simulink library "HIL_GenSet"  (Simulink 7.8)
settings: Solver=ode45  StartTime=0.0  StopTime=10.0  RelTol=1e-3
values from neighbouring files (symbols this model uses):
  Ts = 80e-6    (= 8e-05)    [global_parameters.m]    (also in scopeBuffer.m)
undefined symbols (not defined in the file or in its folder): DiscIntNeverNeededParam, Ts_Power
libraries: simulink x77, powerlib x55, discretizing x28
(part 6 of 9)

== system HIL_GenSet/GenSet_3p5MW_nPID_Manual_RTLAB/Generator with  Primary Controllers/72.5 kva Diesel Engine Speed & Voltage Control fast/IEEE GOVERNOR & DIESEL ENGINE ==
  note: ACTUATOR
  wref (pu) : Inport
  w (pu) : Inport  Port=2
  Reset : Inport  Port=3
  Discrete PID Controller : simulink/Continuous/PID Controller  Controller=PD  TimeDomain=Discrete-time  SampleTime=-1  IntegratorMethod=Forward Euler  FilterMethod=Forward Euler  Form=Parallel  P=1  I=0  D=0.5  N=10000  InitialConditionSource=internal  InitialConditionForIntegrator=0  InitialConditionForFilter=0  ExternalReset=either  ZeroCross=off  LimitOutput=off  UpperSaturationLimit=.5  LowerSaturationLimit=-.5  LinearizeAsGain=off  AntiWindupMode=none  Kb=1  TrackingMode=off  Kt=1  PParamMin=[]  PParamMax=[]  IParamMin=[]  IParamMax=[]  DParamMin=[]  DParamMax=[]  NParamMin=[]  NParamMax=[]  KbParamMin=[]  KbParamMax=[]  KtParamMin=[]  KtParamMax=[]  POutMin=[]  POutMax=[]  IOutMin=[]  IOutMax=[]  DOutMin=[]  DOutMax=[]  NOutMin=[]  NOutMax=[]  KbOutMin=[]  KbOutMax=[]  KtOutMin=[]  KtOutMax=[]  IntegratorOutMin=[]  IntegratorOutMax=[]  FilterOutMin=[]  FilterOutMax=[]  SumOutMin=[]  SumOutMax=[]  SumI1OutMin=[]  SumI1OutMax=[]  SumI2OutMin=[]  SumI2OutMax=[]  SumI3OutMin=[]  SumI3OutMax=[]  SumDOutMin=[]  SumDOutMax=[]  SaturationOutMin=[]  SaturationOutMax=[]  IntegratorContinuousStateAttributes=''  IntegratorStateMustResolveToSignalObject=off  IntegratorRTWStateStorageClass=Auto  FilterContinuousStateAttributes=''  FilterStateMustResolveToSignalObject=off  FilterRTWStateStorageClass=Auto
  Discrete-Time Integrator : DiscreteIntegrator  IntegratorMethod=Integration: Backward Euler  ExternalReset=either  InitialCondition=Pm0  SampleTime=-1  LimitOutput=on  UpperSaturationLimit=Tlim(2)  LowerSaturationLimit=Tlim(1)  ICPrevOutput=DiscIntNeverNeededParam  ICPrevScaledInput=DiscIntNeverNeededParam
  ENGINE Td : TransportDelay  DelayTime=Td  InitialOutput=Pm0  BufferSize=7168
  Gain K : Gain  Gain=K  SaturateOnIntegerOverflow=on  OutDataTypeStr=Inherit: Same as input  ParamDataTypeStr=Inherit: Same as input
  Product : Product  SaturateOnIntegerOverflow=on  InputSameDT=on  OutDataTypeStr=Inherit: Same as first input
  Sum : Sum  Inputs=+-  SaturateOnIntegerOverflow=on  InputSameDT=on  OutDataTypeStr=Inherit: Same as first input
  TF3 : discretizing/Discretized Transfer Fcn  Numerator=1  Denominator=([Ta(3) 1])  AbsTol=auto  SampleTime=Ts  method=zoh  Wc=1
  TF4 : discretizing/Discretized Transfer Fcn  Numerator=([Ta(1) 1])  Denominator=([Ta(2) 1])  AbsTol=auto  SampleTime=Ts  method=zoh  Wc=1
  Pmec (pu) : Outport
  wires:
  Reset/1 -> Discrete PID Controller/2, Discrete-Time Integrator/2
  TF4/1 -> TF3/1
  TF3/1 -> Discrete-Time Integrator/1
  Discrete-Time Integrator/1 -> ENGINE Td/1  "Torque"
  Product/1 -> Pmec (pu)/1
  wref (pu)/1 -> Sum/1
  ENGINE Td/1 -> Product/1
  w (pu)/1 -> Sum/2, Product/2
  Discrete PID Controller/1 -> Gain K/1
  Sum/1 -> Discrete PID Controller/1
  Gain K/1 -> TF4/1

== system HIL_GenSet/GenSet_3p5MW_new_PID_RTLAB/60kW Generator with  Primary Controllers/72.5 kva Diesel Engine Speed & Voltage Control fast/GOVERNOR & DIESEL ENGINE1 ==
  note: ACTUATOR
  wref (pu) : Inport
  w (pu) : Inport  Port=2
  Reset : Inport  Port=3
  Discrete PID Controller : simulink/Continuous/PID Controller  Controller=PD  TimeDomain=Discrete-time  SampleTime=-1  IntegratorMethod=Forward Euler  FilterMethod=Forward Euler  Form=Parallel  P=1  I=0  D=0.5  N=10000  InitialConditionSource=internal  InitialConditionForIntegrator=0  InitialConditionForFilter=0  ExternalReset=either  ZeroCross=off  LimitOutput=off  UpperSaturationLimit=.5  LowerSaturationLimit=-.5  LinearizeAsGain=off  AntiWindupMode=none  Kb=1  TrackingMode=off  Kt=1  PParamMin=[]  PParamMax=[]  IParamMin=[]  IParamMax=[]  DParamMin=[]  DParamMax=[]  NParamMin=[]  NParamMax=[]  KbParamMin=[]  KbParamMax=[]  KtParamMin=[]  KtParamMax=[]  POutMin=[]  POutMax=[]  IOutMin=[]  IOutMax=[]  DOutMin=[]  DOutMax=[]  NOutMin=[]  NOutMax=[]  KbOutMin=[]  KbOutMax=[]  KtOutMin=[]  KtOutMax=[]  IntegratorOutMin=[]  IntegratorOutMax=[]  FilterOutMin=[]  FilterOutMax=[]  SumOutMin=[]  SumOutMax=[]  SumI1OutMin=[]  SumI1OutMax=[]  SumI2OutMin=[]  SumI2OutMax=[]  SumI3OutMin=[]  SumI3OutMax=[]  SumDOutMin=[]  SumDOutMax=[]  SaturationOutMin=[]  SaturationOutMax=[]  IntegratorContinuousStateAttributes=''  IntegratorStateMustResolveToSignalObject=off  IntegratorRTWStateStorageClass=Auto  FilterContinuousStateAttributes=''  FilterStateMustResolveToSignalObject=off  FilterRTWStateStorageClass=Auto
  Discrete-Time Integrator : DiscreteIntegrator  IntegratorMethod=Integration: Backward Euler  ExternalReset=either  InitialCondition=Pm0  SampleTime=Ts_Power  LimitOutput=on  UpperSaturationLimit=Tlim(2)  LowerSaturationLimit=Tlim(1)  ICPrevOutput=DiscIntNeverNeededParam  ICPrevScaledInput=DiscIntNeverNeededParam
  ENGINE Td : TransportDelay  DelayTime=Td  InitialOutput=Pm0  BufferSize=7168
  Gain K : Gain  Gain=K  SaturateOnIntegerOverflow=on  OutDataTypeStr=Inherit: Same as input  ParamDataTypeStr=Inherit: Same as input
  Product : Product  SaturateOnIntegerOverflow=on  InputSameDT=on  OutDataTypeStr=Inherit: Same as first input
  Scope : Scope  NumInputPorts=2
      settings: YMin=-1~-1  YMax=2~2  SaveName=ScopeData20
  Sum : Sum  Inputs=+-  SampleTime=Ts_Power  SaturateOnIntegerOverflow=on  InputSameDT=on  OutDataTypeStr=Inherit: Same as first input
  TF3 : discretizing/Discretized Transfer Fcn  Numerator=1  Denominator=([Ta(3) 1])  AbsTol=auto  SampleTime=Ts_Power  method=zoh  Wc=1
  TF4 : discretizing/Discretized Transfer Fcn  Numerator=([Ta(1) 1])  Denominator=([Ta(2) 1])  AbsTol=auto  SampleTime=Ts_Power  method=zoh  Wc=1
  Pmec (pu) : Outport
  wires:
  Reset/1 -> Discrete PID Controller/2, Discrete-Time Integrator/2
  TF4/1 -> TF3/1
  TF3/1 -> Discrete-Time Integrator/1
  Discrete-Time Integrator/1 -> Scope/2, ENGINE Td/1  "Torque"
  Product/1 -> Scope/1, Pmec (pu)/1
  wref (pu)/1 -> Sum/1
  ENGINE Td/1 -> Product/1
  w (pu)/1 -> Sum/2, Product/2
  Discrete PID Controller/1 -> Gain K/1
  Sum/1 -> Discrete PID Controller/1
  Gain K/1 -> TF4/1

== system HIL_GenSet/GenSet_3p5MW_new_PID_RTLAB/60kW Generator with  Primary Controllers/72.5 kva Diesel Engine Speed & Voltage Control fast/Subsystem ==
  note: link disabled
  note: link disabled
  vref : Inport
  v : Inport  Port=2
  vstab : Inport  Port=3
  Damping kf.s / (tf.s +1) : Subsystem
  Exciter  1 / (te.s + ke) : Subsystem
  Lead Lag Compensator tc.s+1 / tb.s+1 : Subsystem  AncestorBlock=|  mask(Discrete Lead-Lag Controller){T1=tgr(2), T2=tgr(1), V_Init=exc(1)*v0(2)/reg(1), Ts=Ts}
      | powerlib_extras/Discrete 
      | Control Blocks/Discrete
      | Lead-Lag
      mask prompts: T1 "Time constant T1 (s):"; T2 "Time constant T2 (s):"; V_Init "Initial input and output:"; Ts "Sample time (s):"
      mask help:
      | This block implements a discrete lead-lag controller:
      |
      |          1+T1s
      | H(s)= ------
      |          1+T2s
      |
      | States are initialized according to initial input anf output value so that simulation starts in steady state.
      mask init: same as HIL_GenSet/GenSet_3p5MW_RTLAB/60kW Generator with  Primary Controllers/72.5 kva Diesel Engine Speed & Voltage Control fast/Subsystem/Lead Lag Compensator tc.s+1 / tb.s+1
      mask Display: disp('1+T1s\n---\n1+T2s')
  Low Pass Filter 1 / (tr.s +1) (with IC) : Subsystem  AncestorBlock=|  mask(Discrete 1st-Order Filter){FilterType=Lowpass, Tc=tr, Ts=Ts, Initialize=on, Vac_Init=[0 0 60], Vdc_Init=v0(1), PlotResponse=off, param1=[1 500 0.1]}
      | powerlib_extras/Discrete 
      | Control Blocks/Discrete
      | 1st-Order
      | Discrete Filter
      mask prompts: FilterType "Filter Type:"; Tc "Time constant (s):"; Ts "Sample time:"; Initialize "Initialize filter states"; Vac_Init "AC initial input: [ Mag  Phase(degrees)  Freq(Hz) ]"; Vdc_Init "DC Initial input:"; PlotResponse "Plot filter response"; param1 "Frequency range(Hz) : [Start  End  Inc.]"
      mask init: same as HIL_GenSet/GenSet_3p5MW_RTLAB/60kW Generator with  Primary Controllers/72.5 kva Diesel Engine Speed & Voltage Control fast/Subsystem/Low Pass Filter 1 / (tr.s +1) (with IC)
      mask StyleString: popup(Lowpass|Highpass),edit,edit,checkbox,edit,edit,checkbox,edit
      mask CallbackString: |||p4=get_param(gcb,'Initialize');if strcmp(p4,'on');visible={'on','on','on','on','on','on','on',get_param(gcb,'PlotResponse')};else;visible={'on','on','on','on','off','off','on',get_param(gcb,'PlotResponse')};end;set_param(gcb,'MaskVisibilities',visible)|||p7=get_param(gcb,'PlotResponse');if strcmp(p7,'on');visible={'on','on','on','on',get_param(gcb,'Initialize'),get_param(gcb,'Initialize'),'on','on'};else;visible={'on','on','on','on',get_param(gcb,'Initialize'),get_param(gcb,'Initialize'),'on','off'};end;set_param(gcb,'MaskVisibilities',visible)|
      mask Display: plot(X,Y);
  Main Regulator ka / (ta.s +1) : Subsystem
  Sum : Sum  Inputs=++-+-  SaturateOnIntegerOverflow=on  InputSameDT=on  OutDataTypeStr=Inherit: Same as first input
  Unit Delay1 : UnitDelay  SampleTime=Ts
  Unit Delay2 : UnitDelay  X0=v0(2)  SampleTime=Ts
  Vf0 / ka : Constant  Value=v0(2)/reg(1)
  proportional saturation : Subsystem
  Vf1 : Outport  InitialOutput=0
  wires:
  Unit Delay2/1 -> Vf1/1
  Unit Delay1/1 -> Sum/5
  proportional saturation/1(Ef) -> Exciter  1 / (te.s + ke)/1(In)
  Lead Lag Compensator tc.s+1 / tb.s+1/1(Out1) -> Main Regulator ka / (ta.s +1)/1(In)
  Sum/1 -> Lead Lag Compensator tc.s+1 / tb.s+1/1(In1)
  v/1 -> Low Pass Filter 1 / (tr.s +1) (with IC)/1(In)
  vref/1 -> Sum/1
  vstab/1 -> Sum/4
  Low Pass Filter 1 / (tr.s +1) (with IC)/1(Out) -> proportional saturation/2(Vtf), Sum/3
  Vf0 / ka/1 -> Sum/2
  Main Regulator ka / (ta.s +1)/1(Out) -> proportional saturation/1(Efd)
  Damping kf.s / (tf.s +1)/1(Out) -> Unit Delay1/1
  Exciter  1 / (te.s + ke)/1(Out) -> Unit Delay2/1, Damping kf.s / (tf.s +1)/1(In)

== system HIL_GenSet/GenSet_4MW_14kV/Generator with  Primary Controllers/72.5 kva Diesel Engine Speed & Voltage Control fast/IEEE Excitation ==
  note: link disabled
  note: link disabled
  vref : Inport
  v : Inport  Port=2
  vstab : Inport  Port=3
  Damping kf.s / (tf.s +1) : Subsystem
  Exciter  1 / (te.s + ke) : Subsystem
  Lead Lag Compensator tc.s+1 / tb.s+1 : Subsystem  AncestorBlock=|  mask(Discrete Lead-Lag Controller){T1=tgr(2), T2=tgr(1), V_Init=exc(1)*v0(2)/reg(1), Ts=Ts}
      | powerlib_extras/Discrete 
      | Control Blocks/Discrete
      | Lead-Lag
      mask prompts: T1 "Time constant T1 (s):"; T2 "Time constant T2 (s):"; V_Init "Initial input and output:"; Ts "Sample time (s):"
      mask help:
      | This block implements a discrete lead-lag controller:
      |
      |          1+T1s
      | H(s)= ------
      |          1+T2s
      |
      | States are initialized according to initial input anf output value so that simulation starts in steady state.
      mask init: same as HIL_GenSet/GenSet_3p5MW_RTLAB/60kW Generator with  Primary Controllers/72.5 kva Diesel Engine Speed & Voltage Control fast/Subsystem/Lead Lag Compensator tc.s+1 / tb.s+1
      mask Display: disp('1+T1s\n---\n1+T2s')
  Low Pass Filter 1 / (tr.s +1) (with IC) : Subsystem  AncestorBlock=|  mask(Discrete 1st-Order Filter){FilterType=Lowpass, Tc=tr, Ts=Ts, Initialize=on, Vac_Init=[0 0 60], Vdc_Init=v0(1), PlotResponse=off, param1=[1 500 0.1]}
      | powerlib_extras/Discrete 
      | Control Blocks/Discrete
      | 1st-Order
      | Discrete Filter
      mask prompts: FilterType "Filter Type:"; Tc "Time constant (s):"; Ts "Sample time:"; Initialize "Initialize filter states"; Vac_Init "AC initial input: [ Mag  Phase(degrees)  Freq(Hz) ]"; Vdc_Init "DC Initial input:"; PlotResponse "Plot filter response"; param1 "Frequency range(Hz) : [Start  End  Inc.]"
      mask init: same as HIL_GenSet/GenSet_3p5MW_RTLAB/60kW Generator with  Primary Controllers/72.5 kva Diesel Engine Speed & Voltage Control fast/Subsystem/Low Pass Filter 1 / (tr.s +1) (with IC)
      mask StyleString: popup(Lowpass|Highpass),edit,edit,checkbox,edit,edit,checkbox,edit
      mask CallbackString: |||p4=get_param(gcb,'Initialize');if strcmp(p4,'on');visible={'on','on','on','on','on','on','on',get_param(gcb,'PlotResponse')};else;visible={'on','on','on','on','off','off','on',get_param(gcb,'PlotResponse')};end;set_param(gcb,'MaskVisibilities',visible)|||p7=get_param(gcb,'PlotResponse');if strcmp(p7,'on');visible={'on','on','on','on',get_param(gcb,'Initialize'),get_param(gcb,'Initialize'),'on','on'};else;visible={'on','on','on','on',get_param(gcb,'Initialize'),get_param(gcb,'Initialize'),'on','off'};end;set_param(gcb,'MaskVisibilities',visible)|
      mask Display: plot(X,Y);
  Main Regulator ka / (ta.s +1) : Subsystem
  Sum : Sum  Inputs=++-+-  SaturateOnIntegerOverflow=on  InputSameDT=on  OutDataTypeStr=Inherit: Same as first input
  Unit Delay1 : UnitDelay  SampleTime=Ts
  Unit Delay2 : UnitDelay  X0=v0(2)  SampleTime=Ts
  Vf0 / ka : Constant  Value=v0(2)/reg(1)
  proportional saturation : Subsystem
  Vf1 : Outport  InitialOutput=0
  wires:
  Unit Delay2/1 -> Vf1/1
  Unit Delay1/1 -> Sum/5
  proportional saturation/1(Ef) -> Exciter  1 / (te.s + ke)/1(In)
  Lead Lag Compensator tc.s+1 / tb.s+1/1(Out1) -> Main Regulator ka / (ta.s +1)/1(In)
  Sum/1 -> Lead Lag Compensator tc.s+1 / tb.s+1/1(In1)
  v/1 -> Low Pass Filter 1 / (tr.s +1) (with IC)/1(In)
  vref/1 -> Sum/1
  vstab/1 -> Sum/4
  Low Pass Filter 1 / (tr.s +1) (with IC)/1(Out) -> proportional saturation/2(Vtf), Sum/3
  Vf0 / ka/1 -> Sum/2
  Main Regulator ka / (ta.s +1)/1(Out) -> proportional saturation/1(Efd)
  Damping kf.s / (tf.s +1)/1(Out) -> Unit Delay1/1
  Exciter  1 / (te.s + ke)/1(Out) -> Unit Delay2/1, Damping kf.s / (tf.s +1)/1(In)

== system HIL_GenSet/GenSet_4MW_14kV/Generator with  Primary Controllers/72.5 kva Diesel Engine Speed & Voltage Control fast/IEEE GOVERNOR & DIESEL ENGINE ==
  note: ACTUATOR
  wref (pu) : Inport
  w (pu) : Inport  Port=2
  Reset : Inport  Port=3
  Discrete PID Controller : simulink/Continuous/PID Controller  Controller=PD  TimeDomain=Discrete-time  SampleTime=-1  IntegratorMethod=Forward Euler  FilterMethod=Forward Euler  Form=Parallel  P=1  I=0  D=0.5  N=10000  InitialConditionSource=internal  InitialConditionForIntegrator=0  InitialConditionForFilter=0  ExternalReset=either  ZeroCross=off  LimitOutput=off  UpperSaturationLimit=.5  LowerSaturationLimit=-.5  LinearizeAsGain=off  AntiWindupMode=none  Kb=1  TrackingMode=off  Kt=1  PParamMin=[]  PParamMax=[]  IParamMin=[]  IParamMax=[]  DParamMin=[]  DParamMax=[]  NParamMin=[]  NParamMax=[]  KbParamMin=[]  KbParamMax=[]  KtParamMin=[]  KtParamMax=[]  POutMin=[]  POutMax=[]  IOutMin=[]  IOutMax=[]  DOutMin=[]  DOutMax=[]  NOutMin=[]  NOutMax=[]  KbOutMin=[]  KbOutMax=[]  KtOutMin=[]  KtOutMax=[]  IntegratorOutMin=[]  IntegratorOutMax=[]  FilterOutMin=[]  FilterOutMax=[]  SumOutMin=[]  SumOutMax=[]  SumI1OutMin=[]  SumI1OutMax=[]  SumI2OutMin=[]  SumI2OutMax=[]  SumI3OutMin=[]  SumI3OutMax=[]  SumDOutMin=[]  SumDOutMax=[]  SaturationOutMin=[]  SaturationOutMax=[]  IntegratorContinuousStateAttributes=''  IntegratorStateMustResolveToSignalObject=off  IntegratorRTWStateStorageClass=Auto  FilterContinuousStateAttributes=''  FilterStateMustResolveToSignalObject=off  FilterRTWStateStorageClass=Auto
  Discrete-Time Integrator : DiscreteIntegrator  IntegratorMethod=Integration: Backward Euler  ExternalReset=either  InitialCondition=Pm0  SampleTime=-1  LimitOutput=on  UpperSaturationLimit=Tlim(2)  LowerSaturationLimit=Tlim(1)  ICPrevOutput=DiscIntNeverNeededParam  ICPrevScaledInput=DiscIntNeverNeededParam
  ENGINE Td : TransportDelay  DelayTime=Td  InitialOutput=Pm0  BufferSize=7168
  Gain K : Gain  Gain=K  SaturateOnIntegerOverflow=on  OutDataTypeStr=Inherit: Same as input  ParamDataTypeStr=Inherit: Same as input
  Product : Product  SaturateOnIntegerOverflow=on  InputSameDT=on  OutDataTypeStr=Inherit: Same as first input
  Sum : Sum  Inputs=+-  SaturateOnIntegerOverflow=on  InputSameDT=on  OutDataTypeStr=Inherit: Same as first input
  TF3 : discretizing/Discretized Transfer Fcn  Numerator=1  Denominator=([Ta(3) 1])  AbsTol=auto  SampleTime=Ts  method=zoh  Wc=1
  TF4 : discretizing/Discretized Transfer Fcn  Numerator=([Ta(1) 1])  Denominator=([Ta(2) 1])  AbsTol=auto  SampleTime=Ts  method=zoh  Wc=1
  Pmec (pu) : Outport
  wires:
  Reset/1 -> Discrete PID Controller/2, Discrete-Time Integrator/2
  TF4/1 -> TF3/1
  TF3/1 -> Discrete-Time Integrator/1
  Discrete-Time Integrator/1 -> ENGINE Td/1  "Torque"
  Product/1 -> Pmec (pu)/1
  wref (pu)/1 -> Sum/1
  ENGINE Td/1 -> Product/1
  w (pu)/1 -> Sum/2, Product/2
  Discrete PID Controller/1 -> Gain K/1
  Sum/1 -> Discrete PID Controller/1
  Gain K/1 -> TF4/1

== system HIL_GenSet/GenSet_4MW_14kV_07232015/Generator with  Primary Controllers/Diesel Engine Speed & Voltage Control fast/IEEE Excitation ==
  note: link disabled
  note: link disabled
  vref : Inport
  v : Inport  Port=2
  vstab : Inport  Port=3
  Damping kf.s / (tf.s +1) : Subsystem
  Exciter  1 / (te.s + ke) : Subsystem
  Lead Lag Compensator tc.s+1 / tb.s+1 : Subsystem  AncestorBlock=|  mask(Discrete Lead-Lag Controller){T1=tgr(2), T2=tgr(1), V_Init=exc(1)*v0(2)/reg(1), Ts=Ts}
      | powerlib_extras/Discrete 
      | Control Blocks/Discrete
      | Lead-Lag
      mask prompts: T1 "Time constant T1 (s):"; T2 "Time constant T2 (s):"; V_Init "Initial input and output:"; Ts "Sample time (s):"
      mask help:
      | This block implements a discrete lead-lag controller:
      |
      |          1+T1s
      | H(s)= ------
      |          1+T2s
      |
      | States are initialized according to initial input anf output value so that simulation starts in steady state.
      mask init: same as HIL_GenSet/GenSet_3p5MW_RTLAB/60kW Generator with  Primary Controllers/72.5 kva Diesel Engine Speed & Voltage Control fast/Subsystem/Lead Lag Compensator tc.s+1 / tb.s+1
      mask Display: disp('1+T1s\n---\n1+T2s')
  Low Pass Filter 1 / (tr.s +1) (with IC) : Subsystem  AncestorBlock=|  mask(Discrete 1st-Order Filter){FilterType=Lowpass, Tc=tr, Ts=Ts, Initialize=on, Vac_Init=[0 0 60], Vdc_Init=v0(1), PlotResponse=off, param1=[1 500 0.1]}
      | powerlib_extras/Discrete 
      | Control Blocks/Discrete
      | 1st-Order
      | Discrete Filter
      mask prompts: FilterType "Filter Type:"; Tc "Time constant (s):"; Ts "Sample time:"; Initialize "Initialize filter states"; Vac_Init "AC initial input: [ Mag  Phase(degrees)  Freq(Hz) ]"; Vdc_Init "DC Initial input:"; PlotResponse "Plot filter response"; param1 "Frequency range(Hz) : [Start  End  Inc.]"
      mask init: same as HIL_GenSet/GenSet_3p5MW_RTLAB/60kW Generator with  Primary Controllers/72.5 kva Diesel Engine Speed & Voltage Control fast/Subsystem/Low Pass Filter 1 / (tr.s +1) (with IC)
      mask StyleString: popup(Lowpass|Highpass),edit,edit,checkbox,edit,edit,checkbox,edit
      mask CallbackString: |||p4=get_param(gcb,'Initialize');if strcmp(p4,'on');visible={'on','on','on','on','on','on','on',get_param(gcb,'PlotResponse')};else;visible={'on','on','on','on','off','off','on',get_param(gcb,'PlotResponse')};end;set_param(gcb,'MaskVisibilities',visible)|||p7=get_param(gcb,'PlotResponse');if strcmp(p7,'on');visible={'on','on','on','on',get_param(gcb,'Initialize'),get_param(gcb,'Initialize'),'on','on'};else;visible={'on','on','on','on',get_param(gcb,'Initialize'),get_param(gcb,'Initialize'),'on','off'};end;set_param(gcb,'MaskVisibilities',visible)|
      mask Display: plot(X,Y);
  Main Regulator ka / (ta.s +1) : Subsystem
  Sum : Sum  Inputs=++-+-  SaturateOnIntegerOverflow=on  InputSameDT=on  OutDataTypeStr=Inherit: Same as first input
  Unit Delay1 : UnitDelay  SampleTime=Ts
  Unit Delay2 : UnitDelay  X0=v0(2)  SampleTime=Ts
  Vf0 / ka : Constant  Value=v0(2)/reg(1)
  proportional saturation : Subsystem
  Vf1 : Outport  InitialOutput=0
  wires:
  Unit Delay2/1 -> Vf1/1
  Unit Delay1/1 -> Sum/5
  proportional saturation/1(Ef) -> Exciter  1 / (te.s + ke)/1(In)
  Lead Lag Compensator tc.s+1 / tb.s+1/1(Out1) -> Main Regulator ka / (ta.s +1)/1(In)
  Sum/1 -> Lead Lag Compensator tc.s+1 / tb.s+1/1(In1)
  v/1 -> Low Pass Filter 1 / (tr.s +1) (with IC)/1(In)
  vref/1 -> Sum/1
  vstab/1 -> Sum/4
  Low Pass Filter 1 / (tr.s +1) (with IC)/1(Out) -> proportional saturation/2(Vtf), Sum/3
  Vf0 / ka/1 -> Sum/2
  Main Regulator ka / (ta.s +1)/1(Out) -> proportional saturation/1(Efd)
  Damping kf.s / (tf.s +1)/1(Out) -> Unit Delay1/1
  Exciter  1 / (te.s + ke)/1(Out) -> Unit Delay2/1, Damping kf.s / (tf.s +1)/1(In)

== system HIL_GenSet/GenSet_4MW_14kV_07232015/Generator with  Primary Controllers/Diesel Engine Speed & Voltage Control fast/IEEE GOVERNOR & DIESEL ENGINE ==
  note: ACTUATOR
  wref (pu) : Inport
  w (pu) : Inport  Port=2
  Reset : Inport  Port=3
  Discrete PID Controller : simulink/Continuous/PID Controller  Controller=PD  TimeDomain=Discrete-time  SampleTime=-1  IntegratorMethod=Forward Euler  FilterMethod=Forward Euler  Form=Parallel  P=1  I=0  D=0.5  N=10000  InitialConditionSource=internal  InitialConditionForIntegrator=0  InitialConditionForFilter=0  ExternalReset=either  ZeroCross=off  LimitOutput=off  UpperSaturationLimit=.5  LowerSaturationLimit=-.5  LinearizeAsGain=off  AntiWindupMode=none  Kb=1  TrackingMode=off  Kt=1  PParamMin=[]  PParamMax=[]  IParamMin=[]  IParamMax=[]  DParamMin=[]  DParamMax=[]  NParamMin=[]  NParamMax=[]  KbParamMin=[]  KbParamMax=[]  KtParamMin=[]  KtParamMax=[]  POutMin=[]  POutMax=[]  IOutMin=[]  IOutMax=[]  DOutMin=[]  DOutMax=[]  NOutMin=[]  NOutMax=[]  KbOutMin=[]  KbOutMax=[]  KtOutMin=[]  KtOutMax=[]  IntegratorOutMin=[]  IntegratorOutMax=[]  FilterOutMin=[]  FilterOutMax=[]  SumOutMin=[]  SumOutMax=[]  SumI1OutMin=[]  SumI1OutMax=[]  SumI2OutMin=[]  SumI2OutMax=[]  SumI3OutMin=[]  SumI3OutMax=[]  SumDOutMin=[]  SumDOutMax=[]  SaturationOutMin=[]  SaturationOutMax=[]  IntegratorContinuousStateAttributes=''  IntegratorStateMustResolveToSignalObject=off  IntegratorRTWStateStorageClass=Auto  FilterContinuousStateAttributes=''  FilterStateMustResolveToSignalObject=off  FilterRTWStateStorageClass=Auto
  Discrete-Time Integrator : DiscreteIntegrator  IntegratorMethod=Integration: Backward Euler  ExternalReset=either  InitialCondition=Pm0  SampleTime=-1  LimitOutput=on  UpperSaturationLimit=Tlim(2)  LowerSaturationLimit=Tlim(1)  ICPrevOutput=DiscIntNeverNeededParam  ICPrevScaledInput=DiscIntNeverNeededParam
  ENGINE Td : TransportDelay  DelayTime=Td  InitialOutput=Pm0  BufferSize=7168
  Gain K : Gain  Gain=K  SaturateOnIntegerOverflow=on  OutDataTypeStr=Inherit: Same as input  ParamDataTypeStr=Inherit: Same as input
  Product : Product  SaturateOnIntegerOverflow=on  InputSameDT=on  OutDataTypeStr=Inherit: Same as first input
  Sum : Sum  Inputs=+-  SaturateOnIntegerOverflow=on  InputSameDT=on  OutDataTypeStr=Inherit: Same as first input
  TF3 : discretizing/Discretized Transfer Fcn  Numerator=1  Denominator=([Ta(3) 1])  AbsTol=auto  SampleTime=Ts  method=zoh  Wc=1
  TF4 : discretizing/Discretized Transfer Fcn  Numerator=([Ta(1) 1])  Denominator=([Ta(2) 1])  AbsTol=auto  SampleTime=Ts  method=zoh  Wc=1
  Pmec (pu) : Outport
  wires:
  Reset/1 -> Discrete PID Controller/2, Discrete-Time Integrator/2
  TF4/1 -> TF3/1
  TF3/1 -> Discrete-Time Integrator/1
  Discrete-Time Integrator/1 -> ENGINE Td/1  "Torque"
  Product/1 -> Pmec (pu)/1
  wref (pu)/1 -> Sum/1
  ENGINE Td/1 -> Product/1
  w (pu)/1 -> Sum/2, Product/2
  Discrete PID Controller/1 -> Gain K/1
  Sum/1 -> Discrete PID Controller/1
  Gain K/1 -> TF4/1

== system HIL_GenSet/GenSet_4MW_14kV_09022015/Generator with  Primary Controllers/Diesel Engine Speed & Voltage Control fast/IEEE Excitation ==
  note: link disabled
  note: link disabled
  vref : Inport
  v : Inport  Port=2
  vstab : Inport  Port=3
  Damping kf.s / (tf.s +1) : Subsystem
  Exciter  1 / (te.s + ke) : Subsystem
  Lead Lag Compensator tc.s+1 / tb.s+1 : Subsystem  AncestorBlock=|  mask(Discrete Lead-Lag Controller){T1=tgr(2), T2=tgr(1), V_Init=exc(1)*v0(2)/reg(1), Ts=Ts}
      | powerlib_extras/Discrete 
      | Control Blocks/Discrete
      | Lead-Lag
      mask prompts: T1 "Time constant T1 (s):"; T2 "Time constant T2 (s):"; V_Init "Initial input and output:"; Ts "Sample time (s):"
      mask help:
      | This block implements a discrete lead-lag controller:
      |
      |          1+T1s
      | H(s)= ------
      |          1+T2s
      |
      | States are initialized according to initial input anf output value so that simulation starts in steady state.
      mask init: same as HIL_GenSet/GenSet_3p5MW_RTLAB/60kW Generator with  Primary Controllers/72.5 kva Diesel Engine Speed & Voltage Control fast/Subsystem/Lead Lag Compensator tc.s+1 / tb.s+1
      mask Display: disp('1+T1s\n---\n1+T2s')
  Low Pass Filter 1 / (tr.s +1) (with IC) : Subsystem  AncestorBlock=|  mask(Discrete 1st-Order Filter){FilterType=Lowpass, Tc=tr, Ts=Ts, Initialize=on, Vac_Init=[0 0 60], Vdc_Init=v0(1), PlotResponse=off, param1=[1 500 0.1]}
      | powerlib_extras/Discrete 
      | Control Blocks/Discrete
      | 1st-Order
      | Discrete Filter
      mask prompts: FilterType "Filter Type:"; Tc "Time constant (s):"; Ts "Sample time:"; Initialize "Initialize filter states"; Vac_Init "AC initial input: [ Mag  Phase(degrees)  Freq(Hz) ]"; Vdc_Init "DC Initial input:"; PlotResponse "Plot filter response"; param1 "Frequency range(Hz) : [Start  End  Inc.]"
      mask init: same as HIL_GenSet/GenSet_3p5MW_RTLAB/60kW Generator with  Primary Controllers/72.5 kva Diesel Engine Speed & Voltage Control fast/Subsystem/Low Pass Filter 1 / (tr.s +1) (with IC)
      mask StyleString: popup(Lowpass|Highpass),edit,edit,checkbox,edit,edit,checkbox,edit
      mask CallbackString: |||p4=get_param(gcb,'Initialize');if strcmp(p4,'on');visible={'on','on','on','on','on','on','on',get_param(gcb,'PlotResponse')};else;visible={'on','on','on','on','off','off','on',get_param(gcb,'PlotResponse')};end;set_param(gcb,'MaskVisibilities',visible)|||p7=get_param(gcb,'PlotResponse');if strcmp(p7,'on');visible={'on','on','on','on',get_param(gcb,'Initialize'),get_param(gcb,'Initialize'),'on','on'};else;visible={'on','on','on','on',get_param(gcb,'Initialize'),get_param(gcb,'Initialize'),'on','off'};end;set_param(gcb,'MaskVisibilities',visible)|
      mask Display: plot(X,Y);
  Main Regulator ka / (ta.s +1) : Subsystem
  Sum : Sum  Inputs=++-+-  SaturateOnIntegerOverflow=on  InputSameDT=on  OutDataTypeStr=Inherit: Same as first input
  Unit Delay1 : UnitDelay  SampleTime=Ts
  Unit Delay2 : UnitDelay  X0=v0(2)  SampleTime=Ts
  Vf0 / ka : Constant  Value=v0(2)/reg(1)
  proportional saturation : Subsystem
  Vf1 : Outport  InitialOutput=0
  wires:
  Unit Delay2/1 -> Vf1/1
  Unit Delay1/1 -> Sum/5
  proportional saturation/1(Ef) -> Exciter  1 / (te.s + ke)/1(In)
  Lead Lag Compensator tc.s+1 / tb.s+1/1(Out1) -> Main Regulator ka / (ta.s +1)/1(In)
  Sum/1 -> Lead Lag Compensator tc.s+1 / tb.s+1/1(In1)
  v/1 -> Low Pass Filter 1 / (tr.s +1) (with IC)/1(In)
  vref/1 -> Sum/1
  vstab/1 -> Sum/4
  Low Pass Filter 1 / (tr.s +1) (with IC)/1(Out) -> proportional saturation/2(Vtf), Sum/3
  Vf0 / ka/1 -> Sum/2
  Main Regulator ka / (ta.s +1)/1(Out) -> proportional saturation/1(Efd)
  Damping kf.s / (tf.s +1)/1(Out) -> Unit Delay1/1
  Exciter  1 / (te.s + ke)/1(Out) -> Unit Delay2/1, Damping kf.s / (tf.s +1)/1(In)

== system HIL_GenSet/GenSet_4MW_14kV_09022015/Generator with  Primary Controllers/Diesel Engine Speed & Voltage Control fast/IEEE GOVERNOR & DIESEL ENGINE ==
  note: ACTUATOR
  wref (pu) : Inport
  w (pu) : Inport  Port=2
  Reset : Inport  Port=3
  Discrete PID Controller : simulink/Continuous/PID Controller  Controller=PD  TimeDomain=Discrete-time  SampleTime=-1  IntegratorMethod=Forward Euler  FilterMethod=Forward Euler  Form=Parallel  P=1  I=0  D=0.5  N=10000  InitialConditionSource=internal  InitialConditionForIntegrator=0  InitialConditionForFilter=0  ExternalReset=either  ZeroCross=off  LimitOutput=off  UpperSaturationLimit=.5  LowerSaturationLimit=-.5  LinearizeAsGain=off  AntiWindupMode=none  Kb=1  TrackingMode=off  Kt=1  PParamMin=[]  PParamMax=[]  IParamMin=[]  IParamMax=[]  DParamMin=[]  DParamMax=[]  NParamMin=[]  NParamMax=[]  KbParamMin=[]  KbParamMax=[]  KtParamMin=[]  KtParamMax=[]  POutMin=[]  POutMax=[]  IOutMin=[]  IOutMax=[]  DOutMin=[]  DOutMax=[]  NOutMin=[]  NOutMax=[]  KbOutMin=[]  KbOutMax=[]  KtOutMin=[]  KtOutMax=[]  IntegratorOutMin=[]  IntegratorOutMax=[]  FilterOutMin=[]  FilterOutMax=[]  SumOutMin=[]  SumOutMax=[]  SumI1OutMin=[]  SumI1OutMax=[]  SumI2OutMin=[]  SumI2OutMax=[]  SumI3OutMin=[]  SumI3OutMax=[]  SumDOutMin=[]  SumDOutMax=[]  SaturationOutMin=[]  SaturationOutMax=[]  IntegratorContinuousStateAttributes=''  IntegratorStateMustResolveToSignalObject=off  IntegratorRTWStateStorageClass=Auto  FilterContinuousStateAttributes=''  FilterStateMustResolveToSignalObject=off  FilterRTWStateStorageClass=Auto
  Discrete-Time Integrator : DiscreteIntegrator  IntegratorMethod=Integration: Backward Euler  ExternalReset=either  InitialCondition=Pm0  SampleTime=-1  LimitOutput=on  UpperSaturationLimit=Tlim(2)  LowerSaturationLimit=Tlim(1)  ICPrevOutput=DiscIntNeverNeededParam  ICPrevScaledInput=DiscIntNeverNeededParam
  ENGINE Td : TransportDelay  DelayTime=Td  InitialOutput=Pm0  BufferSize=7168
  Gain K : Gain  Gain=K  SaturateOnIntegerOverflow=on  OutDataTypeStr=Inherit: Same as input  ParamDataTypeStr=Inherit: Same as input
  Product : Product  SaturateOnIntegerOverflow=on  InputSameDT=on  OutDataTypeStr=Inherit: Same as first input
  Sum : Sum  Inputs=+-  SaturateOnIntegerOverflow=on  InputSameDT=on  OutDataTypeStr=Inherit: Same as first input
  TF3 : discretizing/Discretized Transfer Fcn  Numerator=1  Denominator=([Ta(3) 1])  AbsTol=auto  SampleTime=Ts  method=zoh  Wc=1
  TF4 : discretizing/Discretized Transfer Fcn  Numerator=([Ta(1) 1])  Denominator=([Ta(2) 1])  AbsTol=auto  SampleTime=Ts  method=zoh  Wc=1
  Pmec (pu) : Outport
  wires:
  Reset/1 -> Discrete PID Controller/2, Discrete-Time Integrator/2
  TF4/1 -> TF3/1
  TF3/1 -> Discrete-Time Integrator/1
  Discrete-Time Integrator/1 -> ENGINE Td/1  "Torque"
  Product/1 -> Pmec (pu)/1
  wref (pu)/1 -> Sum/1
  ENGINE Td/1 -> Product/1
  w (pu)/1 -> Sum/2, Product/2
  Discrete PID Controller/1 -> Gain K/1
  Sum/1 -> Discrete PID Controller/1
  Gain K/1 -> TF4/1

== system HIL_GenSet/GenSet_900kW_07232015/900kW Generator with  Primary Controllers/Diesel Engine Speed & Voltage Control fast/Excitation ==
  note: link disabled
  note: link disabled
  vref : Inport
  v : Inport  Port=2
  vstab : Inport  Port=3
  Damping kf.s / (tf.s +1) : Subsystem
  Exciter  1 / (te.s + ke) : Subsystem
  Lead Lag Compensator tc.s+1 / tb.s+1 : Subsystem  AncestorBlock=|  mask(Discrete Lead-Lag Controller){T1=tgr(2), T2=tgr(1), V_Init=exc(1)*v0(2)/reg(1), Ts=Ts}
      | powerlib_extras/Discrete 
      | Control Blocks/Discrete
      | Lead-Lag
      mask prompts: T1 "Time constant T1 (s):"; T2 "Time constant T2 (s):"; V_Init "Initial input and output:"; Ts "Sample time (s):"
      mask help:
      | This block implements a discrete lead-lag controller:
      |
      |          1+T1s
      | H(s)= ------
      |          1+T2s
      |
      | States are initialized according to initial input anf output value so that simulation starts in steady state.
      mask init: same as HIL_GenSet/GenSet_3p5MW_RTLAB/60kW Generator with  Primary Controllers/72.5 kva Diesel Engine Speed & Voltage Control fast/Subsystem/Lead Lag Compensator tc.s+1 / tb.s+1
      mask Display: disp('1+T1s\n---\n1+T2s')
  Low Pass Filter 1 / (tr.s +1) (with IC) : Subsystem  AncestorBlock=|  mask(Discrete 1st-Order Filter){FilterType=Lowpass, Tc=tr, Ts=Ts, Initialize=on, Vac_Init=[0 0 60], Vdc_Init=v0(1), PlotResponse=off, param1=[1 500 0.1]}
      | powerlib_extras/Discrete 
      | Control Blocks/Discrete
      | 1st-Order
      | Discrete Filter
      mask prompts: FilterType "Filter Type:"; Tc "Time constant (s):"; Ts "Sample time:"; Initialize "Initialize filter states"; Vac_Init "AC initial input: [ Mag  Phase(degrees)  Freq(Hz) ]"; Vdc_Init "DC Initial input:"; PlotResponse "Plot filter response"; param1 "Frequency range(Hz) : [Start  End  Inc.]"
      mask init: same as HIL_GenSet/GenSet_3p5MW_RTLAB/60kW Generator with  Primary Controllers/72.5 kva Diesel Engine Speed & Voltage Control fast/Subsystem/Low Pass Filter 1 / (tr.s +1) (with IC)
      mask StyleString: popup(Lowpass|Highpass),edit,edit,checkbox,edit,edit,checkbox,edit
      mask CallbackString: |||p4=get_param(gcb,'Initialize');if strcmp(p4,'on');visible={'on','on','on','on','on','on','on',get_param(gcb,'PlotResponse')};else;visible={'on','on','on','on','off','off','on',get_param(gcb,'PlotResponse')};end;set_param(gcb,'MaskVisibilities',visible)|||p7=get_param(gcb,'PlotResponse');if strcmp(p7,'on');visible={'on','on','on','on',get_param(gcb,'Initialize'),get_param(gcb,'Initialize'),'on','on'};else;visible={'on','on','on','on',get_param(gcb,'Initialize'),get_param(gcb,'Initialize'),'on','off'};end;set_param(gcb,'MaskVisibilities',visible)|
      mask Display: plot(X,Y);
  Main Regulator ka / (ta.s +1) : Subsystem
  Sum : Sum  Inputs=++-+-  SaturateOnIntegerOverflow=on  InputSameDT=on  OutDataTypeStr=Inherit: Same as first input
  Unit Delay1 : UnitDelay  SampleTime=Ts
  Unit Delay2 : UnitDelay  X0=v0(2)  SampleTime=Ts
  Vf0 / ka : Constant  Value=v0(2)/reg(1)
  proportional saturation : Subsystem
  Vf1 : Outport  InitialOutput=0
  wires:
  Unit Delay2/1 -> Vf1/1
  Unit Delay1/1 -> Sum/5
  proportional saturation/1(Ef) -> Exciter  1 / (te.s + ke)/1(In)
  Lead Lag Compensator tc.s+1 / tb.s+1/1(Out1) -> Main Regulator ka / (ta.s +1)/1(In)
  Sum/1 -> Lead Lag Compensator tc.s+1 / tb.s+1/1(In1)
  v/1 -> Low Pass Filter 1 / (tr.s +1) (with IC)/1(In)
  vref/1 -> Sum/1
  vstab/1 -> Sum/4
  Low Pass Filter 1 / (tr.s +1) (with IC)/1(Out) -> proportional saturation/2(Vtf), Sum/3
  Vf0 / ka/1 -> Sum/2
  Main Regulator ka / (ta.s +1)/1(Out) -> proportional saturation/1(Efd)
  Damping kf.s / (tf.s +1)/1(Out) -> Unit Delay1/1
  Exciter  1 / (te.s + ke)/1(Out) -> Unit Delay2/1, Damping kf.s / (tf.s +1)/1(In)

== system HIL_GenSet/GenSet_900kW_07232015/900kW Generator with  Primary Controllers/Diesel Engine Speed & Voltage Control fast/GOVERNOR & DIESEL ENGINE1 ==
  note: ACTUATOR
  wref (pu) : Inport
  w (pu) : Inport  Port=2
  Reset : Inport  Port=3
  Discrete PID Controller : simulink/Continuous/PID Controller  Controller=PD  TimeDomain=Discrete-time  SampleTime=-1  IntegratorMethod=Forward Euler  FilterMethod=Forward Euler  Form=Parallel  P=1  I=0  D=0.5  N=10000  InitialConditionSource=internal  InitialConditionForIntegrator=0  InitialConditionForFilter=0  ExternalReset=either  ZeroCross=off  LimitOutput=off  UpperSaturationLimit=.5  LowerSaturationLimit=-.5  LinearizeAsGain=off  AntiWindupMode=none  Kb=1  TrackingMode=off  Kt=1  PParamMin=[]  PParamMax=[]  IParamMin=[]  IParamMax=[]  DParamMin=[]  DParamMax=[]  NParamMin=[]  NParamMax=[]  KbParamMin=[]  KbParamMax=[]  KtParamMin=[]  KtParamMax=[]  POutMin=[]  POutMax=[]  IOutMin=[]  IOutMax=[]  DOutMin=[]  DOutMax=[]  NOutMin=[]  NOutMax=[]  KbOutMin=[]  KbOutMax=[]  KtOutMin=[]  KtOutMax=[]  IntegratorOutMin=[]  IntegratorOutMax=[]  FilterOutMin=[]  FilterOutMax=[]  SumOutMin=[]  SumOutMax=[]  SumI1OutMin=[]  SumI1OutMax=[]  SumI2OutMin=[]  SumI2OutMax=[]  SumI3OutMin=[]  SumI3OutMax=[]  SumDOutMin=[]  SumDOutMax=[]  SaturationOutMin=[]  SaturationOutMax=[]  IntegratorContinuousStateAttributes=''  IntegratorStateMustResolveToSignalObject=off  IntegratorRTWStateStorageClass=Auto  FilterContinuousStateAttributes=''  FilterStateMustResolveToSignalObject=off  FilterRTWStateStorageClass=Auto
  Discrete-Time Integrator : DiscreteIntegrator  IntegratorMethod=Integration: Backward Euler  ExternalReset=either  InitialCondition=Pm0  SampleTime=-1  LimitOutput=on  UpperSaturationLimit=Tlim(2)  LowerSaturationLimit=Tlim(1)  ICPrevOutput=DiscIntNeverNeededParam  ICPrevScaledInput=DiscIntNeverNeededParam
  ENGINE Td : TransportDelay  DelayTime=Td  InitialOutput=Pm0  BufferSize=7168
  Gain K : Gain  Gain=K  SaturateOnIntegerOverflow=on  OutDataTypeStr=Inherit: Same as input  ParamDataTypeStr=Inherit: Same as input
  Product : Product  SaturateOnIntegerOverflow=on  InputSameDT=on  OutDataTypeStr=Inherit: Same as first input
  Sum : Sum  Inputs=+-  SaturateOnIntegerOverflow=on  InputSameDT=on  OutDataTypeStr=Inherit: Same as first input
  TF3 : discretizing/Discretized Transfer Fcn  Numerator=1  Denominator=([Ta(3) 1])  AbsTol=auto  SampleTime=Ts  method=zoh  Wc=1
  TF4 : discretizing/Discretized Transfer Fcn  Numerator=([Ta(1) 1])  Denominator=([Ta(2) 1])  AbsTol=auto  SampleTime=Ts  method=zoh  Wc=1
  Pmec (pu) : Outport
  wires:
  Reset/1 -> Discrete PID Controller/2, Discrete-Time Integrator/2
  TF4/1 -> TF3/1
  TF3/1 -> Discrete-Time Integrator/1
  Discrete-Time Integrator/1 -> ENGINE Td/1  "Torque"
  Product/1 -> Pmec (pu)/1
  wref (pu)/1 -> Sum/1
  ENGINE Td/1 -> Product/1
  w (pu)/1 -> Sum/2, Product/2
  Discrete PID Controller/1 -> Gain K/1
  Sum/1 -> Discrete PID Controller/1
  Gain K/1 -> TF4/1

== system HIL_GenSet/GenSet_900kW_RTLAB/Generator with  Primary Controllers1/72.5 kva Diesel Engine Speed & Voltage Control fast/GOVERNOR & DIESEL ENGINE1 ==
  note: ACTUATOR
  wref (pu) : Inport
  w (pu) : Inport  Port=2
  Reset : Inport  Port=3
  Discrete PID Controller : simulink/Continuous/PID Controller  Controller=PD  TimeDomain=Discrete-time  SampleTime=-1  IntegratorMethod=Forward Euler  FilterMethod=Forward Euler  Form=Parallel  P=1  I=0  D=0.5  N=10000  InitialConditionSource=internal  InitialConditionForIntegrator=0  InitialConditionForFilter=0  ExternalReset=either  ZeroCross=off  LimitOutput=off  UpperSaturationLimit=.5  LowerSaturationLimit=-.5  LinearizeAsGain=off  AntiWindupMode=none  Kb=1  TrackingMode=off  Kt=1  PParamMin=[]  PParamMax=[]  IParamMin=[]  IParamMax=[]  DParamMin=[]  DParamMax=[]  NParamMin=[]  NParamMax=[]  KbParamMin=[]  KbParamMax=[]  KtParamMin=[]  KtParamMax=[]  POutMin=[]  POutMax=[]  IOutMin=[]  IOutMax=[]  DOutMin=[]  DOutMax=[]  NOutMin=[]  NOutMax=[]  KbOutMin=[]  KbOutMax=[]  KtOutMin=[]  KtOutMax=[]  IntegratorOutMin=[]  IntegratorOutMax=[]  FilterOutMin=[]  FilterOutMax=[]  SumOutMin=[]  SumOutMax=[]  SumI1OutMin=[]  SumI1OutMax=[]  SumI2OutMin=[]  SumI2OutMax=[]  SumI3OutMin=[]  SumI3OutMax=[]  SumDOutMin=[]  SumDOutMax=[]  SaturationOutMin=[]  SaturationOutMax=[]  IntegratorContinuousStateAttributes=''  IntegratorStateMustResolveToSignalObject=off  IntegratorRTWStateStorageClass=Auto  FilterContinuousStateAttributes=''  FilterStateMustResolveToSignalObject=off  FilterRTWStateStorageClass=Auto
  Discrete-Time Integrator : DiscreteIntegrator  IntegratorMethod=Integration: Backward Euler  ExternalReset=either  InitialCondition=Pm0  SampleTime=-1  LimitOutput=on  UpperSaturationLimit=Tlim(2)  LowerSaturationLimit=Tlim(1)  ICPrevOutput=DiscIntNeverNeededParam  ICPrevScaledInput=DiscIntNeverNeededParam
  ENGINE Td : TransportDelay  DelayTime=Td  InitialOutput=Pm0  BufferSize=7168
  Gain K : Gain  Gain=K  SaturateOnIntegerOverflow=on  OutDataTypeStr=Inherit: Same as input  ParamDataTypeStr=Inherit: Same as input
  Product : Product  SaturateOnIntegerOverflow=on  InputSameDT=on  OutDataTypeStr=Inherit: Same as first input
  Sum : Sum  Inputs=+-  SaturateOnIntegerOverflow=on  InputSameDT=on  OutDataTypeStr=Inherit: Same as first input
  TF3 : discretizing/Discretized Transfer Fcn  Numerator=1  Denominator=([Ta(3) 1])  AbsTol=auto  SampleTime=Ts  method=zoh  Wc=1
  TF4 : discretizing/Discretized Transfer Fcn  Numerator=([Ta(1) 1])  Denominator=([Ta(2) 1])  AbsTol=auto  SampleTime=Ts  method=zoh  Wc=1
  Pmec (pu) : Outport
  wires:
  Reset/1 -> Discrete PID Controller/2, Discrete-Time Integrator/2
  TF4/1 -> TF3/1
  TF3/1 -> Discrete-Time Integrator/1
  Discrete-Time Integrator/1 -> ENGINE Td/1  "Torque"
  Product/1 -> Pmec (pu)/1
  wref (pu)/1 -> Sum/1
  ENGINE Td/1 -> Product/1
  w (pu)/1 -> Sum/2, Product/2
  Discrete PID Controller/1 -> Gain K/1
  Sum/1 -> Discrete PID Controller/1
  Gain K/1 -> TF4/1

== system HIL_GenSet/GenSet_900kW_RTLAB2/60kW Generator with  Primary Controllers/72.5 kva Diesel Engine Speed & Voltage Control fast/GOVERNOR & DIESEL ENGINE1 ==
  note: ACTUATOR
  wref (pu) : Inport
  w (pu) : Inport  Port=2
  Reset : Inport  Port=3
  Discrete PID Controller : simulink/Continuous/PID Controller  Controller=PD  TimeDomain=Discrete-time  SampleTime=-1  IntegratorMethod=Forward Euler  FilterMethod=Forward Euler  Form=Parallel  P=1  I=0  D=0.5  N=10000  InitialConditionSource=internal  InitialConditionForIntegrator=0  InitialConditionForFilter=0  ExternalReset=either  ZeroCross=off  LimitOutput=off  UpperSaturationLimit=.5  LowerSaturationLimit=-.5  LinearizeAsGain=off  AntiWindupMode=none  Kb=1  TrackingMode=off  Kt=1  PParamMin=[]  PParamMax=[]  IParamMin=[]  IParamMax=[]  DParamMin=[]  DParamMax=[]  NParamMin=[]  NParamMax=[]  KbParamMin=[]  KbParamMax=[]  KtParamMin=[]  KtParamMax=[]  POutMin=[]  POutMax=[]  IOutMin=[]  IOutMax=[]  DOutMin=[]  DOutMax=[]  NOutMin=[]  NOutMax=[]  KbOutMin=[]  KbOutMax=[]  KtOutMin=[]  KtOutMax=[]  IntegratorOutMin=[]  IntegratorOutMax=[]  FilterOutMin=[]  FilterOutMax=[]  SumOutMin=[]  SumOutMax=[]  SumI1OutMin=[]  SumI1OutMax=[]  SumI2OutMin=[]  SumI2OutMax=[]  SumI3OutMin=[]  SumI3OutMax=[]  SumDOutMin=[]  SumDOutMax=[]  SaturationOutMin=[]  SaturationOutMax=[]  IntegratorContinuousStateAttributes=''  IntegratorStateMustResolveToSignalObject=off  IntegratorRTWStateStorageClass=Auto  FilterContinuousStateAttributes=''  FilterStateMustResolveToSignalObject=off  FilterRTWStateStorageClass=Auto
  Discrete-Time Integrator : DiscreteIntegrator  IntegratorMethod=Integration: Backward Euler  ExternalReset=either  InitialCondition=Pm0  SampleTime=Ts_Power  LimitOutput=on  UpperSaturationLimit=Tlim(2)  LowerSaturationLimit=Tlim(1)  ICPrevOutput=DiscIntNeverNeededParam  ICPrevScaledInput=DiscIntNeverNeededParam
  ENGINE Td : TransportDelay  DelayTime=Td  InitialOutput=Pm0  BufferSize=7168
  Gain K : Gain  Gain=K  SaturateOnIntegerOverflow=on  OutDataTypeStr=Inherit: Same as input  ParamDataTypeStr=Inherit: Same as input
  Product : Product  SaturateOnIntegerOverflow=on  InputSameDT=on  OutDataTypeStr=Inherit: Same as first input
  Scope : Scope  NumInputPorts=2
      settings: YMin=-1~-1  YMax=2~2  SaveName=ScopeData20
  Sum : Sum  Inputs=+-  SampleTime=Ts_Power  SaturateOnIntegerOverflow=on  InputSameDT=on  OutDataTypeStr=Inherit: Same as first input
  TF3 : discretizing/Discretized Transfer Fcn  Numerator=1  Denominator=([Ta(3) 1])  AbsTol=auto  SampleTime=Ts_Power  method=zoh  Wc=1
  TF4 : discretizing/Discretized Transfer Fcn  Numerator=([Ta(1) 1])  Denominator=([Ta(2) 1])  AbsTol=auto  SampleTime=Ts_Power  method=zoh  Wc=1
  Pmec (pu) : Outport
  wires:
  Reset/1 -> Discrete PID Controller/2, Discrete-Time Integrator/2
  TF4/1 -> TF3/1
  TF3/1 -> Discrete-Time Integrator/1
  Discrete-Time Integrator/1 -> Scope/2, ENGINE Td/1  "Torque"
  Product/1 -> Scope/1, Pmec (pu)/1
  wref (pu)/1 -> Sum/1
  ENGINE Td/1 -> Product/1
  w (pu)/1 -> Sum/2, Product/2
  Discrete PID Controller/1 -> Gain K/1
  Sum/1 -> Discrete PID Controller/1
  Gain K/1 -> TF4/1

== system HIL_GenSet/GenSet_900kW_RTLAB2/60kW Generator with  Primary Controllers/72.5 kva Diesel Engine Speed & Voltage Control fast/Subsystem ==
  note: link disabled
  note: link disabled
  vref : Inport
  v : Inport  Port=2
  vstab : Inport  Port=3
  Damping kf.s / (tf.s +1) : Subsystem
  Exciter  1 / (te.s + ke) : Subsystem
  Lead Lag Compensator tc.s+1 / tb.s+1 : Subsystem  AncestorBlock=|  mask(Discrete Lead-Lag Controller){T1=tgr(2), T2=tgr(1), V_Init=exc(1)*v0(2)/reg(1), Ts=Ts}
      | powerlib_extras/Discrete 
      | Control Blocks/Discrete
      | Lead-Lag
      mask prompts: T1 "Time constant T1 (s):"; T2 "Time constant T2 (s):"; V_Init "Initial input and output:"; Ts "Sample time (s):"
      mask help:
      | This block implements a discrete lead-lag controller:
      |
      |          1+T1s
      | H(s)= ------
      |          1+T2s
      |
      | States are initialized according to initial input anf output value so that simulation starts in steady state.
      mask init: same as HIL_GenSet/GenSet_3p5MW_RTLAB/60kW Generator with  Primary Controllers/72.5 kva Diesel Engine Speed & Voltage Control fast/Subsystem/Lead Lag Compensator tc.s+1 / tb.s+1
      mask Display: disp('1+T1s\n---\n1+T2s')
  Low Pass Filter 1 / (tr.s +1) (with IC) : Subsystem  AncestorBlock=|  mask(Discrete 1st-Order Filter){FilterType=Lowpass, Tc=tr, Ts=Ts, Initialize=on, Vac_Init=[0 0 60], Vdc_Init=v0(1), PlotResponse=off, param1=[1 500 0.1]}
      | powerlib_extras/Discrete 
      | Control Blocks/Discrete
      | 1st-Order
      | Discrete Filter
      mask prompts: FilterType "Filter Type:"; Tc "Time constant (s):"; Ts "Sample time:"; Initialize "Initialize filter states"; Vac_Init "AC initial input: [ Mag  Phase(degrees)  Freq(Hz) ]"; Vdc_Init "DC Initial input:"; PlotResponse "Plot filter response"; param1 "Frequency range(Hz) : [Start  End  Inc.]"
      mask init: same as HIL_GenSet/GenSet_3p5MW_RTLAB/60kW Generator with  Primary Controllers/72.5 kva Diesel Engine Speed & Voltage Control fast/Subsystem/Low Pass Filter 1 / (tr.s +1) (with IC)
      mask StyleString: popup(Lowpass|Highpass),edit,edit,checkbox,edit,edit,checkbox,edit
      mask CallbackString: |||p4=get_param(gcb,'Initialize');if strcmp(p4,'on');visible={'on','on','on','on','on','on','on',get_param(gcb,'PlotResponse')};else;visible={'on','on','on','on','off','off','on',get_param(gcb,'PlotResponse')};end;set_param(gcb,'MaskVisibilities',visible)|||p7=get_param(gcb,'PlotResponse');if strcmp(p7,'on');visible={'on','on','on','on',get_param(gcb,'Initialize'),get_param(gcb,'Initialize'),'on','on'};else;visible={'on','on','on','on',get_param(gcb,'Initialize'),get_param(gcb,'Initialize'),'on','off'};end;set_param(gcb,'MaskVisibilities',visible)|
      mask Display: plot(X,Y);
  Main Regulator ka / (ta.s +1) : Subsystem
  Sum : Sum  Inputs=++-+-  SaturateOnIntegerOverflow=on  InputSameDT=on  OutDataTypeStr=Inherit: Same as first input
  Unit Delay1 : UnitDelay  SampleTime=Ts
  Unit Delay2 : UnitDelay  X0=v0(2)  SampleTime=Ts
  Vf0 / ka : Constant  Value=v0(2)/reg(1)
  proportional saturation : Subsystem
  Vf1 : Outport  InitialOutput=0
  wires:
  Unit Delay2/1 -> Vf1/1
  Unit Delay1/1 -> Sum/5
  proportional saturation/1(Ef) -> Exciter  1 / (te.s + ke)/1(In)
  Lead Lag Compensator tc.s+1 / tb.s+1/1(Out1) -> Main Regulator ka / (ta.s +1)/1(In)
  Sum/1 -> Lead Lag Compensator tc.s+1 / tb.s+1/1(In1)
  v/1 -> Low Pass Filter 1 / (tr.s +1) (with IC)/1(In)
  vref/1 -> Sum/1
  vstab/1 -> Sum/4
  Low Pass Filter 1 / (tr.s +1) (with IC)/1(Out) -> proportional saturation/2(Vtf), Sum/3
  Vf0 / ka/1 -> Sum/2
  Main Regulator ka / (ta.s +1)/1(Out) -> proportional saturation/1(Efd)
  Damping kf.s / (tf.s +1)/1(Out) -> Unit Delay1/1
  Exciter  1 / (te.s + ke)/1(Out) -> Unit Delay2/1, Damping kf.s / (tf.s +1)/1(In)
